simulink model "Project_Model_simulink_version_14_6_2023"  (R2021a)
settings: Solver=FixedStepDiscrete  StartTime=0.0  StopTime=10.0  FixedStep=0.01  RelTol=1e-3
settings Model: Creator=A  LastModifiedBy=A
settings SolverCC: AlgebraicLoopSolver=TrustRegion

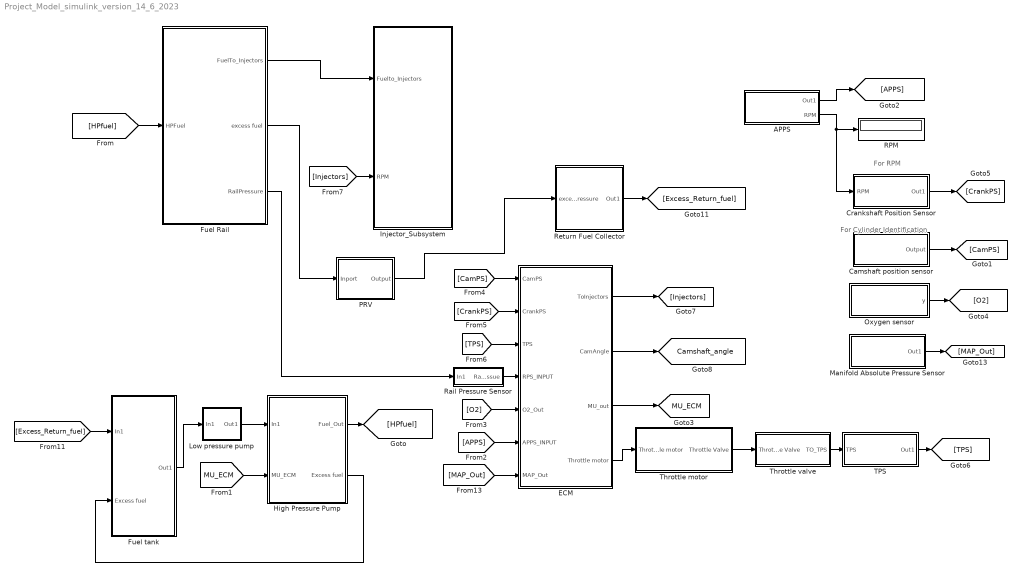
== system Project_Model_simulink_version_14_6_2023 ==
  note: For Cylinder Identification
  note: For RPM
  APPS : Subsystem
  Camshaft position sensor : Subsystem
  Crankshaft Position Sensor : Subsystem
  ECM : Subsystem
  Fuel Rail : Subsystem
  Fuel tank : Subsystem
  High Pressure Pump : Subsystem
  Injector_Subsystem : Subsystem
  Low pressure pump : Subsystem
  Manifold Absolute Pressure Sensor : Subsystem
  Oxygen sensor : Subsystem
  PRV : Subsystem
  RPM : Display
  Rail Pressure Sensor : Subsystem
  Return Fuel Collector : Subsystem
  TPS : Subsystem
  Throttle motor : Subsystem
  Throttle valve : Subsystem
  tag scope: Camshaft_angle=global, MU_ECM=global
  wires:
  Low pressure pump/1(Out1) -> High Pressure Pump/1(In1)
  Fuel tank/1(Out1) -> Low pressure pump/1(In1)
  APPS/1(Out1) -> [APPS]
  [APPS] -> ECM/6(APPS_INPUT)
  ECM/3(MU_out) -> [MU_ECM]
  [O2] -> ECM/5(O2_Out)
  Oxygen sensor/1(y) -> [O2]
  [MU_ECM] -> High Pressure Pump/2(MU_ECM)
  Camshaft position sensor/1(Output) -> [CamPS]
  Fuel Rail/3(RailPressure) -> Rail Pressure Sensor/1(In1)
  Rail Pressure Sensor/1(Rail Pressue) -> ECM/4(RPS_INPUT)
  [CamPS] -> ECM/1(CamPS)
  [CrankPS] -> ECM/2(CrankPS)
  Crankshaft Position Sensor/1(Out1) -> [CrankPS]
  ECM/4(Throttle motor) -> Throttle motor/1(Throttle motor)
  Throttle motor/1(Throttle Valve) -> Throttle valve/1(Throtlle Valve)
  [TPS] -> ECM/3(TPS)
  Fuel Rail/2(excess fuel) -> PRV/1(Inport)
  PRV/1(Output) -> Return Fuel Collector/1(excess rail pressure)
  ECM/1(ToInjectors) -> [Injectors]
  Return Fuel Collector/1(Out1) -> [Excess_Return_fuel]
  [Excess_Return_fuel] -> Fuel tank/1(In1)
  Throttle valve/1(TO_TPS) -> TPS/1(TPS)
  TPS/1(Out1) -> [TPS]
  [MAP_Out] -> ECM/7(MAP_Out)
  Manifold Absolute Pressure Sensor/1(Out1) -> [MAP_Out]
  High Pressure Pump/2(Excess fuel) -> Fuel tank/2(Excess fuel)
  High Pressure Pump/1(Fuel_Out) -> [HPfuel]
  [HPfuel] -> Fuel Rail/1(HPFuel)
  APPS/2(RPM) -> Crankshaft Position Sensor/1(RPM), RPM/1
  Fuel Rail/1(FuelTo_Injectors) -> Injector_Subsystem/1(Fuelto_Injectors)
  [Injectors] -> Injector_Subsystem/2(RPM)
  ECM/2(CamAngle) -> [Camshaft_angle]

== system Project_Model_simulink_version_14_6_2023/APPS ==
  1-D Lookup Table : Lookup_n-D  NumberOfTableDimensions=1  BreakpointsForDimension1=|  BreakpointsForDimension1DataTypeStr=double  Table=|  TableDataTypeStr=double  ExtrapMethod=Clip  InternalRulePriority=Speed  RndMeth=Simplest  InputSameDT=on
      BreakpointsForDimension1=|
      | [8
      | 10
      | 12
      | 14
      | 16
      | 18
      | 20
      | 22
      | 24
      | 26
      | 28
      | 30
      | 32
      | 34
      | 36
      | 38
      | 40
      | 42
      | 44
      | 46
      | 48
      | 50
      | 52
      | 54
      | 56
      | 58
      | 60
      | 62
      | 64
      | 66
      | 68
      | 70
      | 72
      | 74
      | 76
      | 78
      | 80
      | 82
      | 84
      | 86
      | 88
      | 90]
      Table=|
      | [600
      | 730
      | 860
      | 990
      | 1120
      | 1250
      | 1380
      | 1510
      | 1640
      | 1770
      | 1900
      | 2030
      | 2160
      | 2290
      | 2420
      | 2550
      | 2680
      | 2810
      | 2940
      | 3070
      | 3200
      | 3330
      | 3460
      | 3590
      | 3720
      | 3850
      | 3980
      | 4110
      | 4240
      | 4370
      | 4500
      | 4630
      | 4760
      | 4890
      | 5020
      | 5150
      | 5280
      | 5410
      | 5540
      | 5670
      | 5800
      | 6000]
  PedalPositionInDegrees : Constant  Value=11
  Out1 : Outport
  RPM : Outport  Port=2
  tag scope: RPM=global
  wires:
  1-D Lookup Table/1 -> [RPM], RPM/1
  PedalPositionInDegrees/1 -> 1-D Lookup Table/1, Out1/1

== system Project_Model_simulink_version_14_6_2023/Camshaft position sensor ==
  Constant : Constant
  Output : Outport
  wires:
  Constant/1 -> Output/1  "Cam_angle"

== system Project_Model_simulink_version_14_6_2023/Crankshaft Position Sensor ==
  RPM : Inport
  Out1 : Outport
  wires:
  RPM/1 -> Out1/1

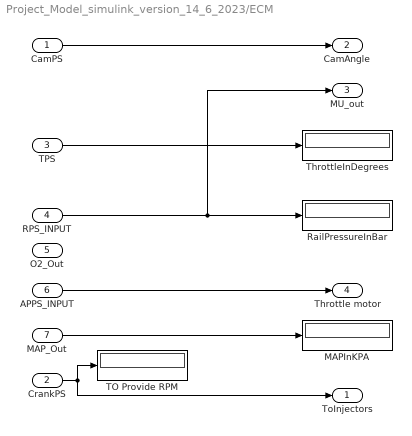
== system Project_Model_simulink_version_14_6_2023/ECM ==
  CamPS : Inport
  CrankPS : Inport  Port=2
  TPS : Inport  Port=3
  RPS_INPUT : Inport  Port=4
  O2_Out : Inport  Port=5
  APPS_INPUT : Inport  Port=6
  MAP_Out : Inport  Port=7
  MAPInKPA : Display
  RailPressureInBar : Display
  TO Provide RPM : Display
  ThrottleInDegrees : Display
  ToInjectors : Outport
  CamAngle : Outport  Port=2
  MU_out : Outport  Port=3
  Throttle motor : Outport  Port=4
  wires:
  CamPS/1 -> CamAngle/1
  APPS_INPUT/1 -> Throttle motor/1
  MAP_Out/1 -> MAPInKPA/1
  TPS/1 -> ThrottleInDegrees/1
  RPS_INPUT/1 -> MU_out/1, RailPressureInBar/1
  CrankPS/1 -> TO Provide RPM/1, ToInjectors/1

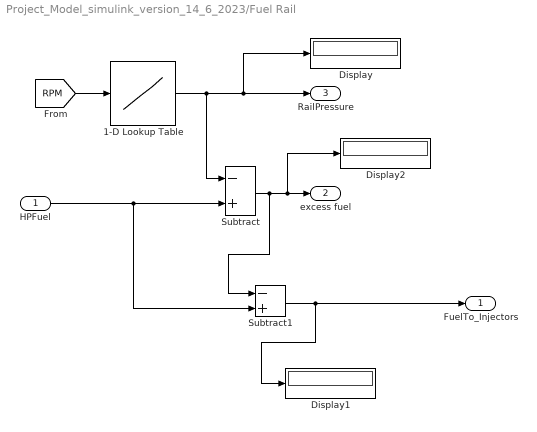
== system Project_Model_simulink_version_14_6_2023/Fuel Rail ==
  HPFuel : Inport
  1-D Lookup Table : Lookup_n-D  NumberOfTableDimensions=1  BreakpointsForDimension1=|  Table=|  InternalRulePriority=Speed  RndMeth=Simplest  InputSameDT=on
      BreakpointsForDimension1=|
      | [600
      | 730
      | 860
      | 990
      | 1120
      | 1250
      | 1380
      | 1510
      | 1640
      | 1770
      | 1900
      | 2030
      | 2160
      | 2290
      | 2420
      | 2550
      | 2680
      | 2810
      | 2940
      | 3070
      | 3200
      | 3330
      | 3460
      | 3590
      | 3720
      | 3850
      | 3980
      | 4110
      | 4240
      | 4370
      | 4500
      | 4630
      | 4760
      | 4890
      | 5020
      | 5150
      | 5280
      | 5410
      | 5540
      | 5670
      | 5800
      | 6000]
      Table=|
      | [300
      | 332
      | 364
      | 396
      | 428
      | 460
      | 492
      | 524
      | 556
      | 588
      | 620
      | 652
      | 684
      | 716
      | 748
      | 780
      | 812
      | 844
      | 876
      | 908
      | 940
      | 972
      | 1004
      | 1036
      | 1068
      | 1100
      | 1132
      | 1164
      | 1196
      | 1228
      | 1260
      | 1292
      | 1324
      | 1356
      | 1388
      | 1420
      | 1452
      | 1484
      | 1516
      | 1548
      | 1580
      | 1600]
  Display : Display
  Display1 : Display
  Display2 : Display
  Subtract : Sum  Inputs=-+
  Subtract1 : Sum  Inputs=-+
  FuelTo_Injectors : Outport
  excess fuel : Outport  Port=2
  RailPressure : Outport  Port=3
  wires:
  1-D Lookup Table/1 -> Subtract/1, Display/1, RailPressure/1
  [RPM] -> 1-D Lookup Table/1
  HPFuel/1 -> Subtract1/2, Subtract/2
  Subtract/1 -> Subtract1/1, Display2/1, excess fuel/1
  Subtract1/1 -> Display1/1, FuelTo_Injectors/1

== system Project_Model_simulink_version_14_6_2023/Fuel tank ==
  In1 : Inport
  Excess fuel : Inport  Port=2
  Constant : Constant
  Out1 : Outport
  wires:
  Constant/1 -> Out1/1

== system Project_Model_simulink_version_14_6_2023/High Pressure Pump ==
  note: rpm=3000
      | rail pressure 902 bar
      | output = 1000 bar
      | difference = 98 bar excess
  In1 : Inport
  MU_ECM : Inport  Port=2
  Display : Display
  Gain : Gain  Gain=160
  Metering Unit : Subsystem
  Fuel_Out : Outport
  Excess fuel : Outport  Port=2
  wires:
  In1/1 -> Gain/1, Display/1
  MU_ECM/1 -> Metering Unit/1(MU_ECM)
  Metering Unit/1(Output) -> Excess fuel/1
  Gain/1 -> Fuel_Out/1

== system Project_Model_simulink_version_14_6_2023/Injector_Subsystem ==
  Fuelto_Injectors : Inport
  RPM : Inport  Port=2
  Injector1 : Subsystem
  Injector2 : Subsystem
  Injector3 : Subsystem
  Injector4 : Subsystem
  wires:
  RPM/1 -> Injector1/1(RPM), Injector2/1(RPM), Injector4/1(RPM), Injector3/1(RPM)
  Fuelto_Injectors/1 -> Injector1/2(HPfuel), Injector2/2(HPfuel), Injector4/2(HPfuel1), Injector3/2(HPfuel)

== system Project_Model_simulink_version_14_6_2023/Low pressure pump ==
  In1 : Inport
  Gain : Gain  Gain=10
  Out1 : Outport
  wires:
  In1/1 -> Gain/1
  Gain/1 -> Out1/1

== system Project_Model_simulink_version_14_6_2023/Manifold Absolute Pressure Sensor ==
  1-D Lookup Table : Lookup_n-D  NumberOfTableDimensions=1  BreakpointsForDimension1=|  Table=|  InternalRulePriority=Speed  RndMeth=Simplest  InputSameDT=on
      BreakpointsForDimension1=|
      | [600
      | 730
      | 860
      | 990
      | 1120
      | 1250
      | 1380
      | 1510
      | 1640
      | 1770
      | 1900
      | 2030
      | 2160
      | 2290
      | 2420
      | 2550
      | 2680
      | 2810
      | 2940
      | 3070
      | 3200
      | 3330
      | 3460
      | 3590
      | 3720
      | 3850
      | 3980
      | 4110
      | 4240
      | 4370
      | 4500
      | 4630
      | 4760
      | 4890
      | 5020
      | 5150
      | 5280
      | 5410
      | 5540
      | 5670
      | 5800
      | 6000]
      Table=|
      | [24
      | 24.2
      | 24.3
      | 24.5
      | 24.6
      | 24.8
      | 24.9
      | 25.1
      | 25.2
      | 25.4
      | 25.5
      | 25.7
      | 25.8
      | 26.0
      | 26.1
      | 26.3
      | 26.4
      | 26.6
      | 26.7
      | 26.9
      | 27.0
      | 27.2
      | 27.3
      | 27.5
      | 27.6
      | 27.8
      | 27.9
      | 28.1
      | 28.2
      | 28.4
      | 28.5
      | 28.7
      | 28.8
      | 29.0
      | 29.1
      | 29.3
      | 29.4
      | 29.5
      | 29.7
      | 29.8
      | 29.9
      | 30]
  Display1 : Display
  Out1 : Outport
  wires:
  1-D Lookup Table/1 -> Out1/1
  [RPM] -> Display1/1, 1-D Lookup Table/1

== system Project_Model_simulink_version_14_6_2023/Oxygen sensor ==
  Constant : Constant
  MATLAB Function : MATLAB Function  TreatAsAtomicUnit=on
  y : Outport
  wires:
  MATLAB Function/1(out) -> y/1
  Constant/1 -> MATLAB Function/1(u)

== system Project_Model_simulink_version_14_6_2023/PRV ==
  Inport : Inport
  Output : Outport
  wires:
  Inport/1 -> Output/1

== system Project_Model_simulink_version_14_6_2023/Rail Pressure Sensor ==
  In1 : Inport
  Rail Pressue : Outport
  wires:
  In1/1 -> Rail Pressue/1

== system Project_Model_simulink_version_14_6_2023/Return Fuel Collector ==
  excess rail pressure : Inport
  Display : Display
  Out1 : Outport
  wires:
  excess rail pressure/1 -> Out1/1, Display/1

== system Project_Model_simulink_version_14_6_2023/TPS ==
  TPS : Inport
  Out1 : Outport
  wires:
  TPS/1 -> Out1/1

== system Project_Model_simulink_version_14_6_2023/Throttle motor ==
  Throttle motor : Inport
  Constant : Constant  Value=pi/3
  Constant1 : Constant
  Integrator : Integrator
  MATLAB Function : MATLAB Function  TreatAsAtomicUnit=on
  Mux : Mux  Inputs=2
  accelerator_pedal : Subsystem
  engine_controll_unit : Subsystem
  feedback_sensor : Subsystem
      settings: PortSchema="{\"entries\":[{\"content\":{\"sides\":[{\"content\":{\"connectorIds\":[\"Out1\"]},\"type\":\"ConnectorPlacement.EquallySpacedRectSide\",\"uuid\":\"fe640009-eb11-44be-8596-49d62a5beec8\"},{\"content\":{\"connectorIds\":[\"In1\"],\"side\":\"RIGHT\"},\"type\":\"ConnectorPlacement.EquallySpacedRectSide\",\"uuid\":\"55096441-78fe-4501-a0f7-12f27b21a046\"},{\"content\":{\"connectorIds\":[],\"side\":\"TOP\"},\"type\":\"ConnectorPlacement.EquallySpacedRectSide\",\"uuid\":\"eb36a32d-1c61-4111-82c5-835a656f9bf6\"}]},\"type\":\"ConnectorPlacement.EquallySpacedConnector\",\"uuid\":\"24611814-9bea-49d8-8ce5-1a9dc2d12b43\"}],\"packageUris\":[\"http://schema.mathworks.com/mf0/Connector/R2020b\"],\"version\":\"1.0\"}"
  throttle_system : Subsystem
  Throttle Valve : Outport
  wires:
  Throttle motor/1 -> Throttle Valve/1
  MATLAB Function/1(y) -> accelerator_pedal/1(angel)
  Mux/1 -> MATLAB Function/1(u)
  engine_controll_unit/1(duty) -> throttle_system/2(duty)
  throttle_system/1(theta) -> feedback_sensor/1(throttle_angle)
  engine_controll_unit/2(direction) -> throttle_system/1(direction)
  Constant1/1 -> Integrator/1
  accelerator_pedal/1(voltage) -> engine_controll_unit/1(pedal_volt)
  feedback_sensor/1(throttle_voltage) -> engine_controll_unit/2(throttle _volt)
  Integrator/1 -> Mux/1
  Constant/1 -> Mux/2

== system Project_Model_simulink_version_14_6_2023/Throttle valve ==
  Throtlle Valve : Inport
  TO_TPS : Outport
  wires:
  Throtlle Valve/1 -> TO_TPS/1

== system Project_Model_simulink_version_14_6_2023/High Pressure Pump/Metering Unit ==
  note: if fuel pressure in rail is as per the required in specific rpm then duty cycle is 15 % if pressure is more duty cylce will increase to 20 % until pressure in rail is as per required
  MU_ECM : Inport
  Output : Outport
  wires:
  MU_ECM/1 -> Output/1

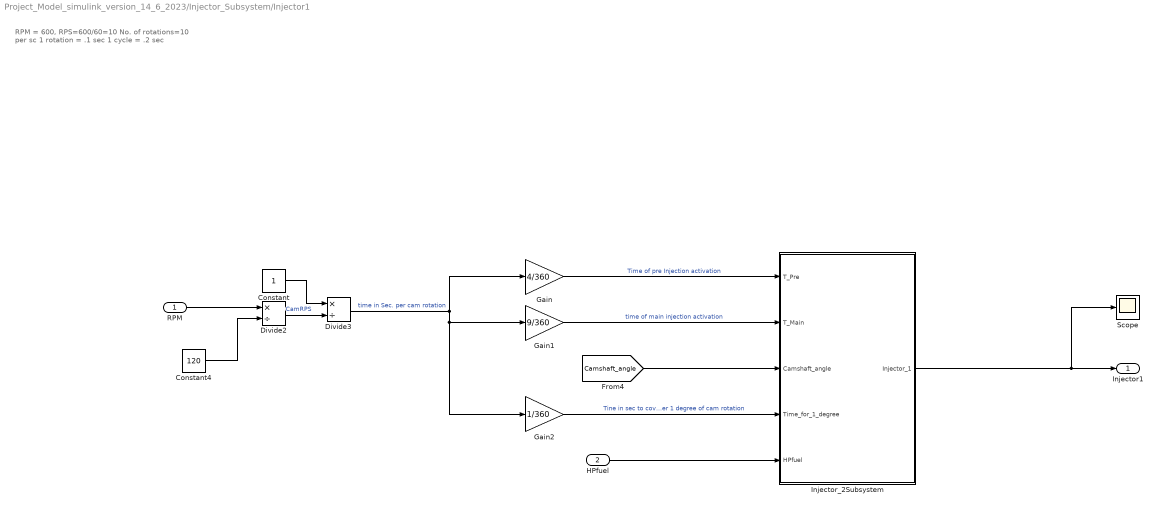
== system Project_Model_simulink_version_14_6_2023/Injector_Subsystem/Injector1 ==
  note: RPM = 600,
      | RPS=600/60=10
      | No. of rotations=10 per sc
      | 1 rotation = .1 sec
      | 1 cycle = .2 sec
  RPM : Inport
  HPfuel : Inport  Port=2
  Constant : Constant
  Constant4 : Constant  Value=120
  Divide2 : Product  Inputs=*/
  Divide3 : Product  Inputs=*/
  Gain : Gain  Gain=4/360
  Gain1 : Gain  Gain=9/360
  Gain2 : Gain  Gain=1/360
  Injector_2Subsystem : Subsystem  TreatAsAtomicUnit=on
  Scope : Scope
  Injector1 : Outport
  wires:
  Gain2/1 -> Injector_2Subsystem/4(Time_for_1_degree)  "Tine in sec to cover 1 degree of cam rotation"
  Gain/1 -> Injector_2Subsystem/1(T_Pre)  "Time of pre Injection activation"
  RPM/1 -> Divide2/1
  Divide3/1 -> Gain/1, Gain2/1, Gain1/1  "time in Sec. per cam rotation"
  Injector_2Subsystem/1(Injector_1) -> Scope/1, Injector1/1
  Divide2/1 -> Divide3/2  "CamRPS"
  [Camshaft_angle] -> Injector_2Subsystem/3(Camshaft_angle)
  HPfuel/1 -> Injector_2Subsystem/5(HPfuel)
  Gain1/1 -> Injector_2Subsystem/2(T_Main)  "time of main injection activation"
  Constant/1 -> Divide3/1
  Constant4/1 -> Divide2/2

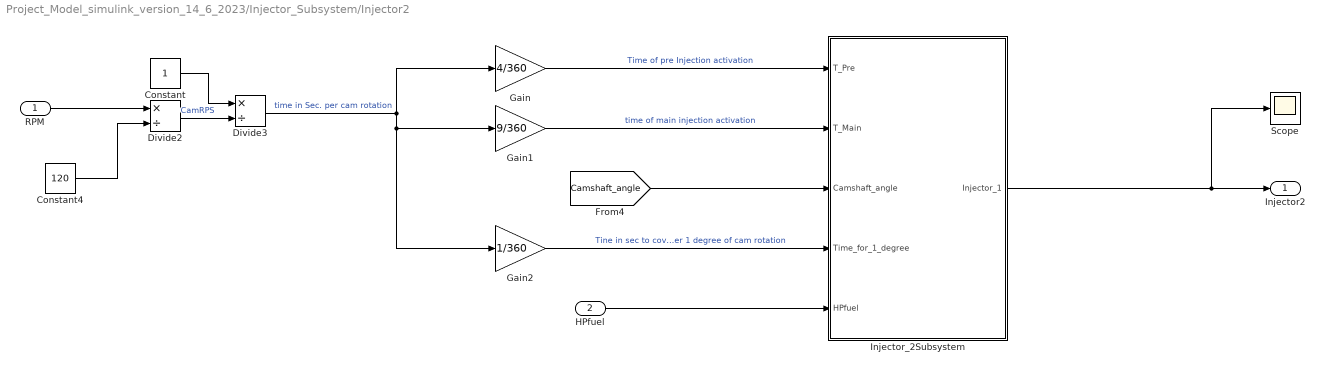
== system Project_Model_simulink_version_14_6_2023/Injector_Subsystem/Injector2 ==
  RPM : Inport
  HPfuel : Inport  Port=2
  Constant : Constant
  Constant4 : Constant  Value=120
  Divide2 : Product  Inputs=*/
  Divide3 : Product  Inputs=*/
  Gain : Gain  Gain=4/360
  Gain1 : Gain  Gain=9/360
  Gain2 : Gain  Gain=1/360
  Injector_2Subsystem : Subsystem  TreatAsAtomicUnit=on
  Scope : Scope
  Injector2 : Outport
  wires:
  Gain2/1 -> Injector_2Subsystem/4(Time_for_1_degree)  "Tine in sec to cover 1 degree of cam rotation"
  Gain/1 -> Injector_2Subsystem/1(T_Pre)  "Time of pre Injection activation"
  RPM/1 -> Divide2/1
  Divide3/1 -> Gain/1, Gain2/1, Gain1/1  "time in Sec. per cam rotation"
  Injector_2Subsystem/1(Injector_1) -> Scope/1, Injector2/1
  Divide2/1 -> Divide3/2  "CamRPS"
  [Camshaft_angle] -> Injector_2Subsystem/3(Camshaft_angle)
  HPfuel/1 -> Injector_2Subsystem/5(HPfuel)
  Gain1/1 -> Injector_2Subsystem/2(T_Main)  "time of main injection activation"
  Constant/1 -> Divide3/1
  Constant4/1 -> Divide2/2

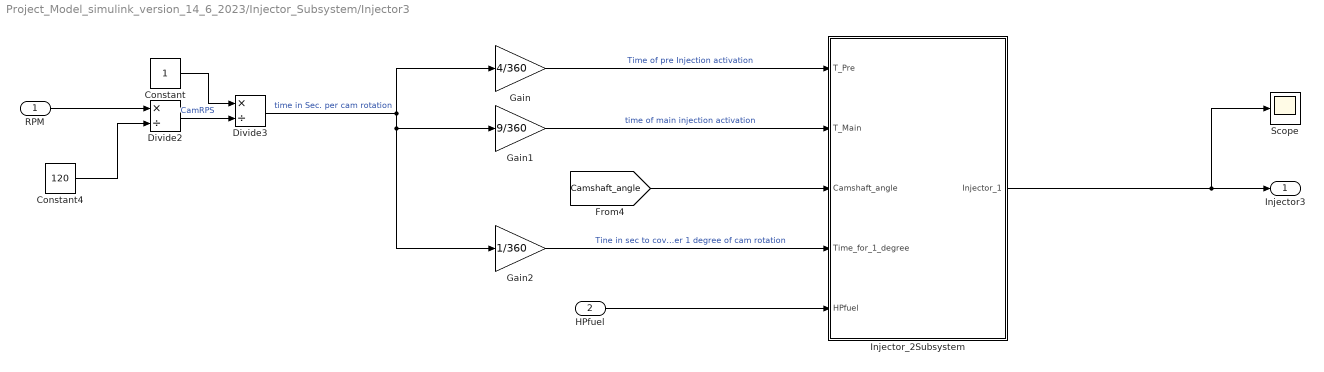
== system Project_Model_simulink_version_14_6_2023/Injector_Subsystem/Injector3 ==
  RPM : Inport
  HPfuel : Inport  Port=2
  Constant : Constant
  Constant4 : Constant  Value=120
  Divide2 : Product  Inputs=*/
  Divide3 : Product  Inputs=*/
  Gain : Gain  Gain=4/360
  Gain1 : Gain  Gain=9/360
  Gain2 : Gain  Gain=1/360
  Injector_2Subsystem : Subsystem  TreatAsAtomicUnit=on
  Scope : Scope
  Injector3 : Outport
  wires:
  Injector_2Subsystem/1(Injector_1) -> Scope/1, Injector3/1
  [Camshaft_angle] -> Injector_2Subsystem/3(Camshaft_angle)
  Gain2/1 -> Injector_2Subsystem/4(Time_for_1_degree)  "Tine in sec to cover 1 degree of cam rotation"
  HPfuel/1 -> Injector_2Subsystem/5(HPfuel)
  Divide3/1 -> Gain/1, Gain2/1, Gain1/1  "time in Sec. per cam rotation"
  Divide2/1 -> Divide3/2  "CamRPS"
  Gain/1 -> Injector_2Subsystem/1(T_Pre)  "Time of pre Injection activation"
  Constant/1 -> Divide3/1
  Constant4/1 -> Divide2/2
  RPM/1 -> Divide2/1
  Gain1/1 -> Injector_2Subsystem/2(T_Main)  "time of main injection activation"

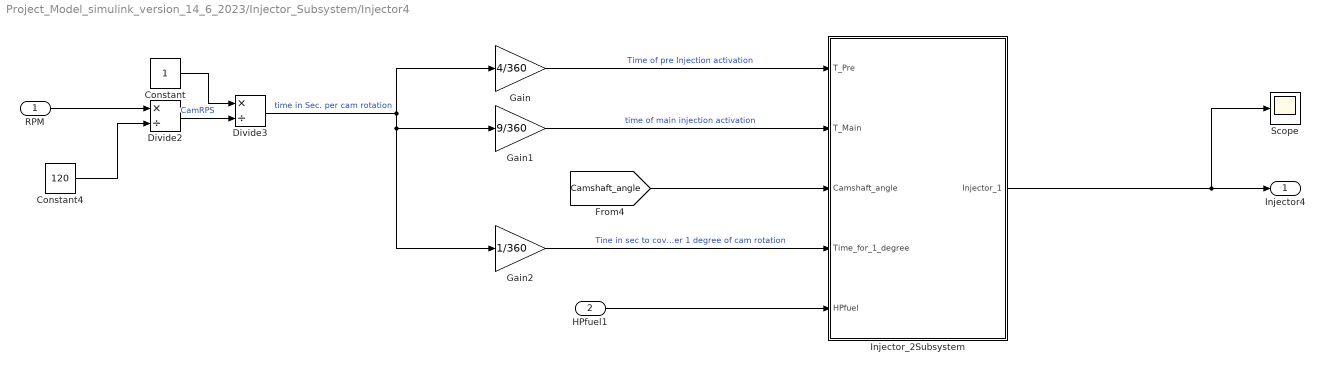
== system Project_Model_simulink_version_14_6_2023/Injector_Subsystem/Injector4 ==
  RPM : Inport
  HPfuel1 : Inport  Port=2
  Constant : Constant
  Constant4 : Constant  Value=120
  Divide2 : Product  Inputs=*/
  Divide3 : Product  Inputs=*/
  Gain : Gain  Gain=4/360
  Gain1 : Gain  Gain=9/360
  Gain2 : Gain  Gain=1/360
  Injector_2Subsystem : Subsystem  TreatAsAtomicUnit=on
  Scope : Scope
  Injector4 : Outport
  wires:
  Gain2/1 -> Injector_2Subsystem/4(Time_for_1_degree)  "Tine in sec to cover 1 degree of cam rotation"
  Gain/1 -> Injector_2Subsystem/1(T_Pre)  "Time of pre Injection activation"
  RPM/1 -> Divide2/1
  Divide3/1 -> Gain/1, Gain2/1, Gain1/1  "time in Sec. per cam rotation"
  Injector_2Subsystem/1(Injector_1) -> Scope/1, Injector4/1
  Divide2/1 -> Divide3/2  "CamRPS"
  [Camshaft_angle] -> Injector_2Subsystem/3(Camshaft_angle)
  HPfuel1/1 -> Injector_2Subsystem/5(HPfuel)
  Gain1/1 -> Injector_2Subsystem/2(T_Main)  "time of main injection activation"
  Constant/1 -> Divide3/1
  Constant4/1 -> Divide2/2

== system Project_Model_simulink_version_14_6_2023/Throttle motor/accelerator_pedal ==
  angel : Inport
  1-D Lookup Table : Lookup_n-D  NumberOfTableDimensions=1  BreakpointsForDimension1=[0 90]  Table=[0.5 4.5]  InternalRulePriority=Speed  RndMeth=Simplest  InputSameDT=on
  Gain : Gain  Gain=180/pi
  voltage : Outport
  wires:
  1-D Lookup Table/1 -> voltage/1
  Gain/1 -> 1-D Lookup Table/1
  angel/1 -> Gain/1

== system Project_Model_simulink_version_14_6_2023/Throttle motor/engine_controll_unit ==
  pedal_volt : Inport
  throttle _volt : Inport  Port=2
  Add : Sum  Inputs=+-
  Subsystem : Subsystem
  duty : Outport
  direction : Outport  Port=2
  wires:
  Add/1 -> Subsystem/1(In1)
  pedal_volt/1 -> Add/1
  throttle _volt/1 -> Add/2
  Subsystem/1(Out1) -> duty/1
  Subsystem/2(Out2) -> direction/1

== system Project_Model_simulink_version_14_6_2023/Throttle motor/feedback_sensor ==
  throttle_angle : Inport
  Subsystem : Subsystem
  throttle_voltage : Outport
  wires:
  throttle_angle/1 -> Subsystem/1(angle)
  Subsystem/1(voltage) -> throttle_voltage/1

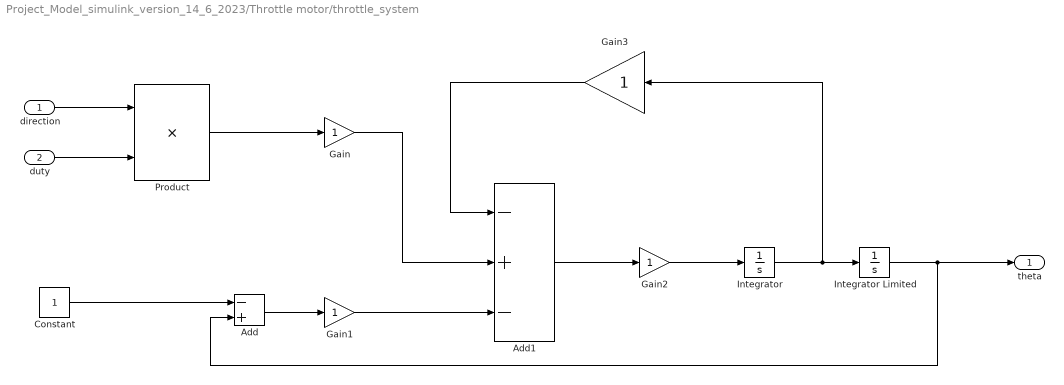
== system Project_Model_simulink_version_14_6_2023/Throttle motor/throttle_system ==
  direction : Inport
  duty : Inport  Port=2
  Add : Sum  Inputs=-+
  Add1 : Sum  Inputs=-+-
  Constant : Constant
  Gain{,1..3} (4 alike) : Gain
  Integrator : Integrator
  Integrator Limited : Integrator  LimitOutput=on  UpperSaturationLimit=pi/2  LowerSaturationLimit=0
  Product : Product
  theta : Outport
  wires:
  direction/1 -> Product/1
  duty/1 -> Product/2
  Product/1 -> Gain/1
  Add/1 -> Gain1/1
  Gain/1 -> Add1/2
  Gain1/1 -> Add1/3
  Constant/1 -> Add/1
  Gain2/1 -> Integrator/1
  Add1/1 -> Gain2/1
  Integrator/1 -> Gain3/1, Integrator Limited/1
  Integrator Limited/1 -> Add/2, theta/1
  Gain3/1 -> Add1/1

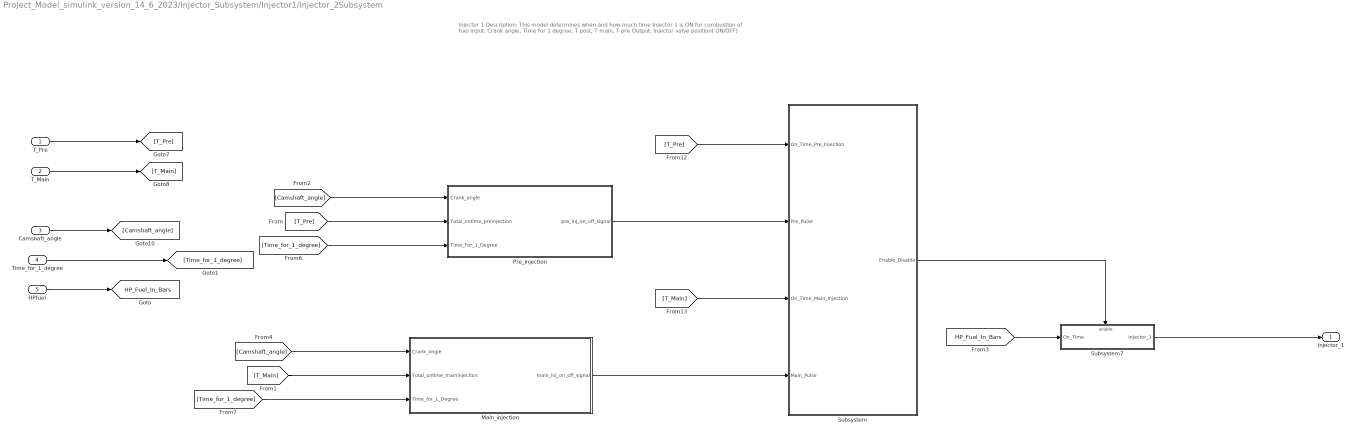
== system Project_Model_simulink_version_14_6_2023/Injector_Subsystem/Injector1/Injector_2Subsystem ==
  note: Injector 1
      | Description: This model determines when and how much time Injector 1 is ON for combustion of fuel
      | Input: Crank angle, TIme for 1 degree, T post, T main, T pre
      | Output: Injector valve position( ON/OFF)
  T_Pre : Inport
  T_Main : Inport  Port=2
  Camshaft_angle : Inport  Port=3
  Time_for_1_degree : Inport  Port=4
  HPfuel : Inport  Port=5
  Main_injection : Subsystem  TreatAsAtomicUnit=on
  Pre_injection : Subsystem  TreatAsAtomicUnit=on
  Subsystem : Subsystem
  Subsystem7 : Subsystem
  Injector_1 : Outport
  tag scope: HP_Fuel_In_Bars=global
  wires:
  T_Pre/1 -> [T_Pre]
  T_Main/1 -> [T_Main]
  Time_for_1_degree/1 -> [Time_for_1_degree]
  [Time_for_1_degree] -> Main_injection/3(Time_for_1_Degree)
  [T_Main] -> Main_injection/2(Total_ontime_maininjection)
  [Camshaft_angle] -> Main_injection/1(Crank_angle)
  [Time_for_1_degree] -> Pre_injection/3(Time_For_1_Degree)
  [Camshaft_angle] -> Pre_injection/1(Crank_angle)
  [T_Pre] -> Pre_injection/2(Total_ontime_preinjection)
  Subsystem/1(Enable_Disable) -> Subsystem7/Enable
  Subsystem7/1(Injector_1) -> Injector_1/1
  [T_Pre] -> Subsystem/1(On_Time_Pre_Injection)
  [T_Main] -> Subsystem/3(On_Time_Main_Injection)
  Main_injection/1(main_inj_on_off_signal) -> Subsystem/4(Main_Pulse)
  Pre_injection/1(pre_inj_on_off_signal) -> Subsystem/2(Pre_Pulse)
  [HP_Fuel_In_Bars] -> Subsystem7/1(On_Time)
  HPfuel/1 -> [HP_Fuel_In_Bars]
  Camshaft_angle/1 -> [Camshaft_angle]

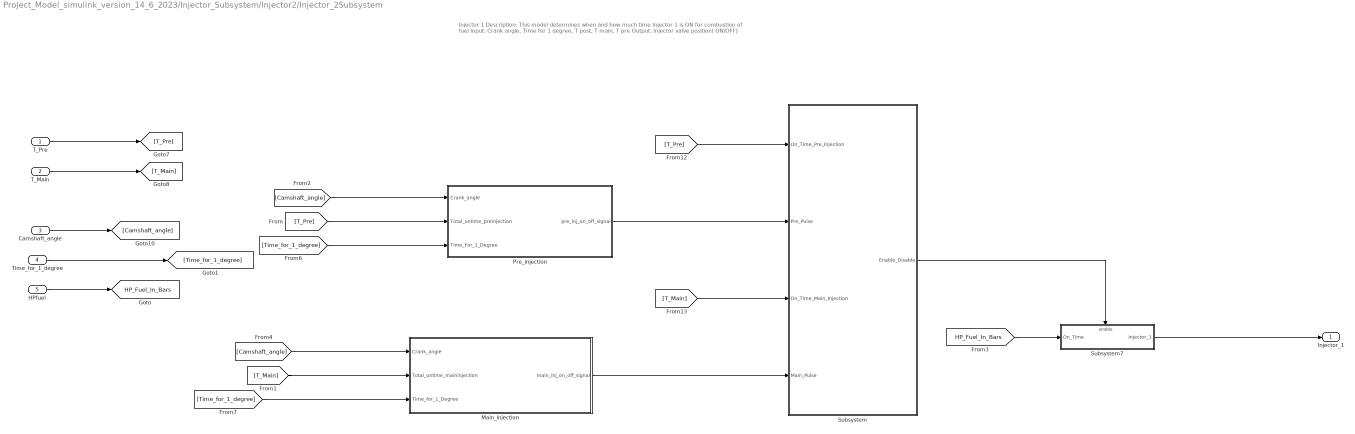
== system Project_Model_simulink_version_14_6_2023/Injector_Subsystem/Injector2/Injector_2Subsystem ==
  note: Injector 1
      | Description: This model determines when and how much time Injector 1 is ON for combustion of fuel
      | Input: Crank angle, TIme for 1 degree, T post, T main, T pre
      | Output: Injector valve position( ON/OFF)
  T_Pre : Inport
  T_Main : Inport  Port=2
  Camshaft_angle : Inport  Port=3
  Time_for_1_degree : Inport  Port=4
  HPfuel : Inport  Port=5
  Main_injection : Subsystem  TreatAsAtomicUnit=on
  Pre_injection : Subsystem  TreatAsAtomicUnit=on
  Subsystem : Subsystem
  Subsystem7 : Subsystem
  Injector_1 : Outport
  tag scope: HP_Fuel_In_Bars=global
  wires:
  T_Pre/1 -> [T_Pre]
  T_Main/1 -> [T_Main]
  Time_for_1_degree/1 -> [Time_for_1_degree]
  [Time_for_1_degree] -> Main_injection/3(Time_for_1_Degree)
  [T_Main] -> Main_injection/2(Total_ontime_maininjection)
  [Camshaft_angle] -> Main_injection/1(Crank_angle)
  [Time_for_1_degree] -> Pre_injection/3(Time_For_1_Degree)
  [Camshaft_angle] -> Pre_injection/1(Crank_angle)
  [T_Pre] -> Pre_injection/2(Total_ontime_preinjection)
  Subsystem/1(Enable_Disable) -> Subsystem7/Enable
  Subsystem7/1(Injector_1) -> Injector_1/1
  [T_Pre] -> Subsystem/1(On_Time_Pre_Injection)
  [T_Main] -> Subsystem/3(On_Time_Main_Injection)
  Main_injection/1(main_inj_on_off_signal) -> Subsystem/4(Main_Pulse)
  Pre_injection/1(pre_inj_on_off_signal) -> Subsystem/2(Pre_Pulse)
  [HP_Fuel_In_Bars] -> Subsystem7/1(On_Time)
  HPfuel/1 -> [HP_Fuel_In_Bars]
  Camshaft_angle/1 -> [Camshaft_angle]

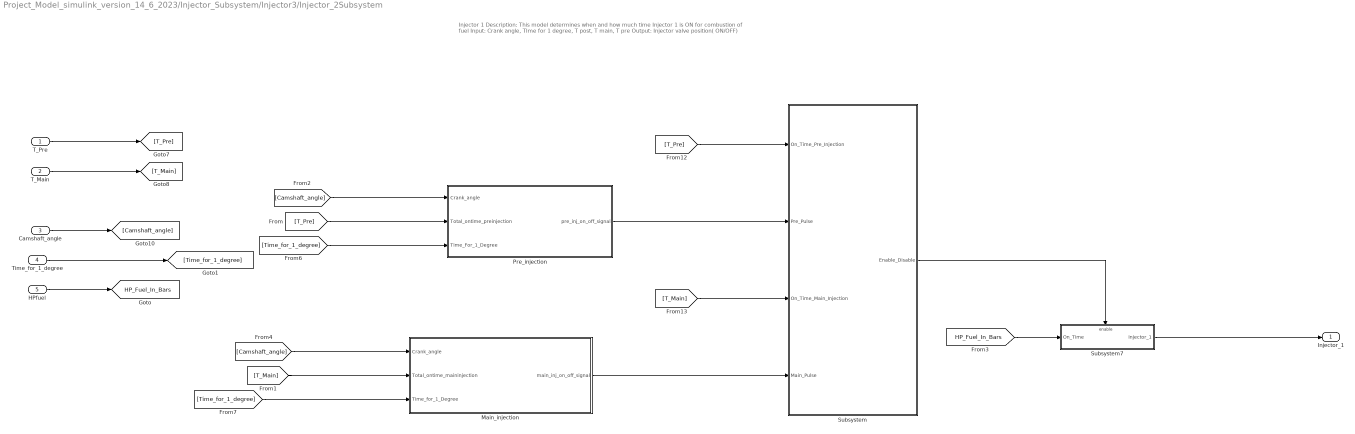
== system Project_Model_simulink_version_14_6_2023/Injector_Subsystem/Injector3/Injector_2Subsystem ==
  note: Injector 1
      | Description: This model determines when and how much time Injector 1 is ON for combustion of fuel
      | Input: Crank angle, TIme for 1 degree, T post, T main, T pre
      | Output: Injector valve position( ON/OFF)
  T_Pre : Inport
  T_Main : Inport  Port=2
  Camshaft_angle : Inport  Port=3
  Time_for_1_degree : Inport  Port=4
  HPfuel : Inport  Port=5
  Main_injection : Subsystem  TreatAsAtomicUnit=on
  Pre_injection : Subsystem  TreatAsAtomicUnit=on
  Subsystem : Subsystem
  Subsystem7 : Subsystem
  Injector_1 : Outport
  tag scope: HP_Fuel_In_Bars=global
  wires:
  T_Pre/1 -> [T_Pre]
  T_Main/1 -> [T_Main]
  Time_for_1_degree/1 -> [Time_for_1_degree]
  [Time_for_1_degree] -> Main_injection/3(Time_for_1_Degree)
  [T_Main] -> Main_injection/2(Total_ontime_maininjection)
  [Camshaft_angle] -> Main_injection/1(Crank_angle)
  [Time_for_1_degree] -> Pre_injection/3(Time_For_1_Degree)
  [Camshaft_angle] -> Pre_injection/1(Crank_angle)
  [T_Pre] -> Pre_injection/2(Total_ontime_preinjection)
  Subsystem/1(Enable_Disable) -> Subsystem7/Enable
  Subsystem7/1(Injector_1) -> Injector_1/1
  [T_Pre] -> Subsystem/1(On_Time_Pre_Injection)
  [T_Main] -> Subsystem/3(On_Time_Main_Injection)
  Main_injection/1(main_inj_on_off_signal) -> Subsystem/4(Main_Pulse)
  Pre_injection/1(pre_inj_on_off_signal) -> Subsystem/2(Pre_Pulse)
  [HP_Fuel_In_Bars] -> Subsystem7/1(On_Time)
  HPfuel/1 -> [HP_Fuel_In_Bars]
  Camshaft_angle/1 -> [Camshaft_angle]

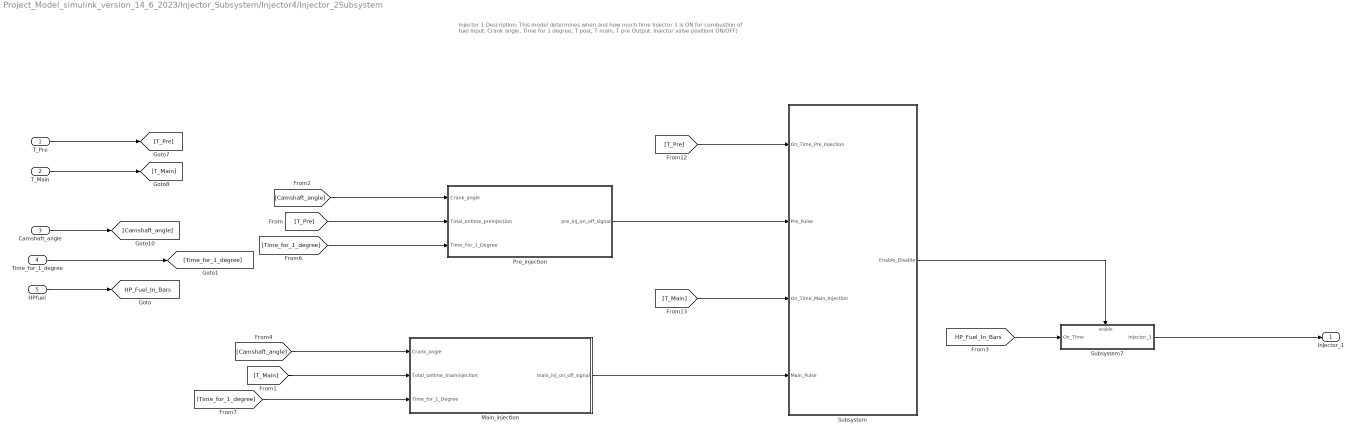
== system Project_Model_simulink_version_14_6_2023/Injector_Subsystem/Injector4/Injector_2Subsystem ==
  note: Injector 1
      | Description: This model determines when and how much time Injector 1 is ON for combustion of fuel
      | Input: Crank angle, TIme for 1 degree, T post, T main, T pre
      | Output: Injector valve position( ON/OFF)
  T_Pre : Inport
  T_Main : Inport  Port=2
  Camshaft_angle : Inport  Port=3
  Time_for_1_degree : Inport  Port=4
  HPfuel : Inport  Port=5
  Main_injection : Subsystem  TreatAsAtomicUnit=on
  Pre_injection : Subsystem  TreatAsAtomicUnit=on
  Subsystem : Subsystem
  Subsystem7 : Subsystem
  Injector_1 : Outport
  tag scope: HP_Fuel_In_Bars=global
  wires:
  T_Pre/1 -> [T_Pre]
  T_Main/1 -> [T_Main]
  Time_for_1_degree/1 -> [Time_for_1_degree]
  [Time_for_1_degree] -> Main_injection/3(Time_for_1_Degree)
  [T_Main] -> Main_injection/2(Total_ontime_maininjection)
  [Camshaft_angle] -> Main_injection/1(Crank_angle)
  [Time_for_1_degree] -> Pre_injection/3(Time_For_1_Degree)
  [Camshaft_angle] -> Pre_injection/1(Crank_angle)
  [T_Pre] -> Pre_injection/2(Total_ontime_preinjection)
  Subsystem/1(Enable_Disable) -> Subsystem7/Enable
  Subsystem7/1(Injector_1) -> Injector_1/1
  [T_Pre] -> Subsystem/1(On_Time_Pre_Injection)
  [T_Main] -> Subsystem/3(On_Time_Main_Injection)
  Main_injection/1(main_inj_on_off_signal) -> Subsystem/4(Main_Pulse)
  Pre_injection/1(pre_inj_on_off_signal) -> Subsystem/2(Pre_Pulse)
  [HP_Fuel_In_Bars] -> Subsystem7/1(On_Time)
  HPfuel/1 -> [HP_Fuel_In_Bars]
  Camshaft_angle/1 -> [Camshaft_angle]

== system Project_Model_simulink_version_14_6_2023/Throttle motor/engine_controll_unit/Subsystem ==
  In1 : Inport
  Abs : Abs
  Constant : Constant
  Constant1 : Constant  Value=-1
  Saturation : Saturate
  Switch : Switch
  Out1 : Outport
  Out2 : Outport  Port=2
  wires:
  Abs/1 -> Saturation/1
  In1/1 -> Switch/2, Abs/1
  Constant/1 -> Switch/1
  Constant1/1 -> Switch/3
  Saturation/1 -> Out1/1
  Switch/1 -> Out2/1

== system Project_Model_simulink_version_14_6_2023/Throttle motor/feedback_sensor/Subsystem ==
  angle : Inport
  1-D Lookup Table : Lookup_n-D  NumberOfTableDimensions=1  BreakpointsForDimension1=[0 90]  Table=[0.5 4.5]  InternalRulePriority=Speed  RndMeth=Simplest  InputSameDT=on
  Gain : Gain  Gain=180/pi
  voltage : Outport
  wires:
  1-D Lookup Table/1 -> voltage/1
  Gain/1 -> 1-D Lookup Table/1
  angle/1 -> Gain/1

== system Project_Model_simulink_version_14_6_2023/Injector_Subsystem/Injector1/Injector_2Subsystem/Main_injection ==
  Crank_angle : Inport  OutDataTypeStr=single
  Total_ontime_maininjection : Inport  Port=2  OutDataTypeStr=single
  Time_for_1_Degree : Inport  Port=3  OutDataTypeStr=single
  Add : Sum  AccumDataTypeStr=single
      settings: AttributesFormatString=AccumDataTypeStr=%<AccumDataTypeStr>
  Divide : Product  Inputs=*/  OutDataTypeStr=single
  Logical Operator : Logic  AllPortsSameDT=off  OutDataTypeStr=boolean
  Main_Inj_trg_angle_inj1 : Constant  Value=180
  Main_Inj_trg_angle_inj2 : Constant  Value=180
  Relational Operator : RelationalOperator  OutDataTypeStr=boolean  RndMeth=Simplest
  Relational Operator1 : RelationalOperator  Operator=<=  OutDataTypeStr=boolean  RndMeth=Simplest
  main_inj_on_off_signal : Outport  VectorParamsAs1DForOutWhenUnconnected=off
  wires:
  Logical Operator/1 -> main_inj_on_off_signal/1  "main_inj_on_off_signal"
  Time_for_1_Degree/1 -> Divide/2
  Relational Operator/1 -> Logical Operator/1
  Main_Inj_trg_angle_inj2/1 -> Add/1
  Add/1 -> Relational Operator1/2  "Total_On_Degree"
  Crank_angle/1 -> Relational Operator1/1, Relational Operator/1
  Main_Inj_trg_angle_inj1/1 -> Relational Operator/2
  Relational Operator1/1 -> Logical Operator/2
  Total_ontime_maininjection/1 -> Divide/1
  Divide/1 -> Add/2

== system Project_Model_simulink_version_14_6_2023/Injector_Subsystem/Injector1/Injector_2Subsystem/Pre_injection ==
  Crank_angle : Inport  OutDataTypeStr=single
  Total_ontime_preinjection : Inport  Port=2  OutDataTypeStr=single
  Time_For_1_Degree : Inport  Port=3  OutDataTypeStr=single
  Add : Sum  AccumDataTypeStr=single
      settings: AttributesFormatString=AccumDataTypeStr=%<AccumDataTypeStr>
  Divide : Product  Inputs=*/  OutDataTypeStr=single
  Logical Operator : Logic  AllPortsSameDT=off  OutDataTypeStr=boolean
  Pre_Inj_trg_angle_inj1 : Constant  Value=175
  Pre_Inj_trg_angle_inj2 : Constant  Value=175
  Relational Operator : RelationalOperator  OutDataTypeStr=boolean  RndMeth=Simplest
  Relational Operator1 : RelationalOperator  Operator=<=  OutDataTypeStr=boolean  RndMeth=Simplest
  pre_inj_on_off_signal : Outport  VectorParamsAs1DForOutWhenUnconnected=off
  wires:
  Divide/1 -> Add/2
  Relational Operator1/1 -> Logical Operator/2
  Pre_Inj_trg_angle_inj1/1 -> Relational Operator/2  "<Trigger_angle>"
  Total_ontime_preinjection/1 -> Divide/1
  Add/1 -> Relational Operator1/2  "Total_On_Degree"
  Pre_Inj_trg_angle_inj2/1 -> Add/1  "<Trigger_angle>"
  Time_For_1_Degree/1 -> Divide/2
  Relational Operator/1 -> Logical Operator/1
  Crank_angle/1 -> Relational Operator1/1, Relational Operator/1
  Logical Operator/1 -> pre_inj_on_off_signal/1  "pre_inj_on_off_signal"

== system Project_Model_simulink_version_14_6_2023/Injector_Subsystem/Injector1/Injector_2Subsystem/Subsystem ==
  note: Subsystem
      | Description: Integrates Pre, Main, Post Injection to single output
      | Input: On time for pre Injection, On time for main Injection, On time for post Injection, Pre Pulse, Main Pulse, Post Pulse
      | Output: On time for Injection
  On_Time_Pre_Injection : Inport
  Pre_Pulse : Inport  Port=2
  On_Time_Main_Injection : Inport  Port=3
  Main_Pulse : Inport  Port=4
  Constant : Constant  Value=0
  Switch1 : Switch  Criteria=u2 ~= 0
  Switch2 : Switch  Criteria=u2 ~= 0
  Enable_Disable : Outport  VectorParamsAs1DForOutWhenUnconnected=off
  wires:
  Main_Pulse/1 -> [main1], Switch2/2
  On_Time_Main_Injection/1 -> Switch2/1
  Pre_Pulse/1 -> Switch1/2, [pre1]
  On_Time_Pre_Injection/1 -> Switch1/1
  Switch1/1 -> Enable_Disable/1  "On_Time_Injection"
  Constant/1 -> Switch2/3  "constant"
  Switch2/1 -> Switch1/3

== system Project_Model_simulink_version_14_6_2023/Injector_Subsystem/Injector1/Injector_2Subsystem/Subsystem7 ==
  note: Pulse for Injector 1
      | Description: Give signal to Injector 1
      | Input: Re rounding constant
      | Output: Pulse to Injector 1
  On_Time : Inport
  Enable : EnablePort  StatesWhenEnabling=reset  PropagateVarSize=During execution
  Injector_1 : Outport  OutDataTypeStr=boolean  VectorParamsAs1DForOutWhenUnconnected=off
  wires:
  On_Time/1 -> Injector_1/1  "HP_fuel_in_Bars"

== system Project_Model_simulink_version_14_6_2023/Injector_Subsystem/Injector2/Injector_2Subsystem/Main_injection ==
  Crank_angle : Inport  OutDataTypeStr=single
  Total_ontime_maininjection : Inport  Port=2  OutDataTypeStr=single
  Time_for_1_Degree : Inport  Port=3  OutDataTypeStr=single
  Add : Sum  AccumDataTypeStr=single
      settings: AttributesFormatString=AccumDataTypeStr=%<AccumDataTypeStr>
  Divide : Product  Inputs=*/  OutDataTypeStr=single
  Logical Operator : Logic  AllPortsSameDT=off  OutDataTypeStr=boolean
  Main_Inj_trg_angle_inj1 : Constant  Value=180
  Main_Inj_trg_angle_inj2 : Constant  Value=180
  Relational Operator : RelationalOperator  OutDataTypeStr=boolean  RndMeth=Simplest
  Relational Operator1 : RelationalOperator  Operator=<=  OutDataTypeStr=boolean  RndMeth=Simplest
  main_inj_on_off_signal : Outport  VectorParamsAs1DForOutWhenUnconnected=off
  wires:
  Logical Operator/1 -> main_inj_on_off_signal/1  "main_inj_on_off_signal"
  Time_for_1_Degree/1 -> Divide/2
  Relational Operator/1 -> Logical Operator/1
  Main_Inj_trg_angle_inj2/1 -> Add/1
  Add/1 -> Relational Operator1/2  "Total_On_Degree"
  Crank_angle/1 -> Relational Operator1/1, Relational Operator/1
  Main_Inj_trg_angle_inj1/1 -> Relational Operator/2
  Relational Operator1/1 -> Logical Operator/2
  Total_ontime_maininjection/1 -> Divide/1
  Divide/1 -> Add/2

== system Project_Model_simulink_version_14_6_2023/Injector_Subsystem/Injector2/Injector_2Subsystem/Pre_injection ==
  Crank_angle : Inport  OutDataTypeStr=single
  Total_ontime_preinjection : Inport  Port=2  OutDataTypeStr=single
  Time_For_1_Degree : Inport  Port=3  OutDataTypeStr=single
  Add : Sum  AccumDataTypeStr=single
      settings: AttributesFormatString=AccumDataTypeStr=%<AccumDataTypeStr>
  Divide : Product  Inputs=*/  OutDataTypeStr=single
  Logical Operator : Logic  AllPortsSameDT=off  OutDataTypeStr=boolean
  Pre_Inj_trg_angle_inj1 : Constant  Value=175
  Pre_Inj_trg_angle_inj2 : Constant  Value=175
  Relational Operator : RelationalOperator  OutDataTypeStr=boolean  RndMeth=Simplest
  Relational Operator1 : RelationalOperator  Operator=<=  OutDataTypeStr=boolean  RndMeth=Simplest
  pre_inj_on_off_signal : Outport  VectorParamsAs1DForOutWhenUnconnected=off
  wires:
  Divide/1 -> Add/2
  Relational Operator1/1 -> Logical Operator/2
  Pre_Inj_trg_angle_inj1/1 -> Relational Operator/2  "<Trigger_angle>"
  Total_ontime_preinjection/1 -> Divide/1
  Add/1 -> Relational Operator1/2  "Total_On_Degree"
  Pre_Inj_trg_angle_inj2/1 -> Add/1  "<Trigger_angle>"
  Time_For_1_Degree/1 -> Divide/2
  Relational Operator/1 -> Logical Operator/1
  Crank_angle/1 -> Relational Operator1/1, Relational Operator/1
  Logical Operator/1 -> pre_inj_on_off_signal/1  "pre_inj_on_off_signal"

== system Project_Model_simulink_version_14_6_2023/Injector_Subsystem/Injector2/Injector_2Subsystem/Subsystem ==
  note: Subsystem
      | Description: Integrates Pre, Main, Post Injection to single output
      | Input: On time for pre Injection, On time for main Injection, On time for post Injection, Pre Pulse, Main Pulse, Post Pulse
      | Output: On time for Injection
  On_Time_Pre_Injection : Inport
  Pre_Pulse : Inport  Port=2
  On_Time_Main_Injection : Inport  Port=3
  Main_Pulse : Inport  Port=4
  Constant : Constant  Value=0
  Switch1 : Switch  Criteria=u2 ~= 0
  Switch2 : Switch  Criteria=u2 ~= 0
  Enable_Disable : Outport  VectorParamsAs1DForOutWhenUnconnected=off
  wires:
  Main_Pulse/1 -> [main1], Switch2/2
  On_Time_Main_Injection/1 -> Switch2/1
  Pre_Pulse/1 -> Switch1/2, [pre1]
  On_Time_Pre_Injection/1 -> Switch1/1
  Switch1/1 -> Enable_Disable/1  "On_Time_Injection"
  Constant/1 -> Switch2/3  "constant"
  Switch2/1 -> Switch1/3

== system Project_Model_simulink_version_14_6_2023/Injector_Subsystem/Injector2/Injector_2Subsystem/Subsystem7 ==
  note: Pulse for Injector 1
      | Description: Give signal to Injector 1
      | Input: Re rounding constant
      | Output: Pulse to Injector 1
  On_Time : Inport
  Enable : EnablePort  StatesWhenEnabling=reset  PropagateVarSize=During execution
  Injector_1 : Outport  OutDataTypeStr=boolean  VectorParamsAs1DForOutWhenUnconnected=off
  wires:
  On_Time/1 -> Injector_1/1  "HP_fuel_in_Bars"

== system Project_Model_simulink_version_14_6_2023/Injector_Subsystem/Injector3/Injector_2Subsystem/Main_injection ==
  Crank_angle : Inport  OutDataTypeStr=single
  Total_ontime_maininjection : Inport  Port=2  OutDataTypeStr=single
  Time_for_1_Degree : Inport  Port=3  OutDataTypeStr=single
  Add : Sum  AccumDataTypeStr=single
      settings: AttributesFormatString=AccumDataTypeStr=%<AccumDataTypeStr>
  Divide : Product  Inputs=*/  OutDataTypeStr=single
  Logical Operator : Logic  AllPortsSameDT=off  OutDataTypeStr=boolean
  Main_Inj_trg_angle_inj1 : Constant  Value=180
  Main_Inj_trg_angle_inj2 : Constant  Value=180
  Relational Operator : RelationalOperator  OutDataTypeStr=boolean  RndMeth=Simplest
  Relational Operator1 : RelationalOperator  Operator=<=  OutDataTypeStr=boolean  RndMeth=Simplest
  main_inj_on_off_signal : Outport  VectorParamsAs1DForOutWhenUnconnected=off
  wires:
  Logical Operator/1 -> main_inj_on_off_signal/1  "main_inj_on_off_signal"
  Time_for_1_Degree/1 -> Divide/2
  Relational Operator/1 -> Logical Operator/1
  Main_Inj_trg_angle_inj2/1 -> Add/1
  Add/1 -> Relational Operator1/2  "Total_On_Degree"
  Crank_angle/1 -> Relational Operator1/1, Relational Operator/1
  Main_Inj_trg_angle_inj1/1 -> Relational Operator/2
  Relational Operator1/1 -> Logical Operator/2
  Total_ontime_maininjection/1 -> Divide/1
  Divide/1 -> Add/2

== system Project_Model_simulink_version_14_6_2023/Injector_Subsystem/Injector3/Injector_2Subsystem/Pre_injection ==
  Crank_angle : Inport  OutDataTypeStr=single
  Total_ontime_preinjection : Inport  Port=2  OutDataTypeStr=single
  Time_For_1_Degree : Inport  Port=3  OutDataTypeStr=single
  Add : Sum  AccumDataTypeStr=single
      settings: AttributesFormatString=AccumDataTypeStr=%<AccumDataTypeStr>
  Divide : Product  Inputs=*/  OutDataTypeStr=single
  Logical Operator : Logic  AllPortsSameDT=off  OutDataTypeStr=boolean
  Pre_Inj_trg_angle_inj1 : Constant  Value=175
  Pre_Inj_trg_angle_inj2 : Constant  Value=175
  Relational Operator : RelationalOperator  OutDataTypeStr=boolean  RndMeth=Simplest
  Relational Operator1 : RelationalOperator  Operator=<=  OutDataTypeStr=boolean  RndMeth=Simplest
  pre_inj_on_off_signal : Outport  VectorParamsAs1DForOutWhenUnconnected=off
  wires:
  Divide/1 -> Add/2
  Relational Operator1/1 -> Logical Operator/2
  Pre_Inj_trg_angle_inj1/1 -> Relational Operator/2  "<Trigger_angle>"
  Total_ontime_preinjection/1 -> Divide/1
  Add/1 -> Relational Operator1/2  "Total_On_Degree"
  Pre_Inj_trg_angle_inj2/1 -> Add/1  "<Trigger_angle>"
  Time_For_1_Degree/1 -> Divide/2
  Relational Operator/1 -> Logical Operator/1
  Crank_angle/1 -> Relational Operator1/1, Relational Operator/1
  Logical Operator/1 -> pre_inj_on_off_signal/1  "pre_inj_on_off_signal"

== system Project_Model_simulink_version_14_6_2023/Injector_Subsystem/Injector3/Injector_2Subsystem/Subsystem ==
  note: Subsystem
      | Description: Integrates Pre, Main, Post Injection to single output
      | Input: On time for pre Injection, On time for main Injection, On time for post Injection, Pre Pulse, Main Pulse, Post Pulse
      | Output: On time for Injection
  On_Time_Pre_Injection : Inport
  Pre_Pulse : Inport  Port=2
  On_Time_Main_Injection : Inport  Port=3
  Main_Pulse : Inport  Port=4
  Constant : Constant  Value=0
  Switch1 : Switch  Criteria=u2 ~= 0
  Switch2 : Switch  Criteria=u2 ~= 0
  Enable_Disable : Outport  VectorParamsAs1DForOutWhenUnconnected=off
  wires:
  Main_Pulse/1 -> [main1], Switch2/2
  On_Time_Main_Injection/1 -> Switch2/1
  Pre_Pulse/1 -> Switch1/2, [pre1]
  On_Time_Pre_Injection/1 -> Switch1/1
  Switch1/1 -> Enable_Disable/1  "On_Time_Injection"
  Constant/1 -> Switch2/3  "constant"
  Switch2/1 -> Switch1/3

== system Project_Model_simulink_version_14_6_2023/Injector_Subsystem/Injector3/Injector_2Subsystem/Subsystem7 ==
  note: Pulse for Injector 1
      | Description: Give signal to Injector 1
      | Input: Re rounding constant
      | Output: Pulse to Injector 1
  On_Time : Inport
  Enable : EnablePort  StatesWhenEnabling=reset  PropagateVarSize=During execution
  Injector_1 : Outport  OutDataTypeStr=boolean  VectorParamsAs1DForOutWhenUnconnected=off
  wires:
  On_Time/1 -> Injector_1/1  "HP_fuel_in_Bars"

== system Project_Model_simulink_version_14_6_2023/Injector_Subsystem/Injector4/Injector_2Subsystem/Main_injection ==
  Crank_angle : Inport  OutDataTypeStr=single
  Total_ontime_maininjection : Inport  Port=2  OutDataTypeStr=single
  Time_for_1_Degree : Inport  Port=3  OutDataTypeStr=single
  Add : Sum  AccumDataTypeStr=single
      settings: AttributesFormatString=AccumDataTypeStr=%<AccumDataTypeStr>
  Divide : Product  Inputs=*/  OutDataTypeStr=single
  Logical Operator : Logic  AllPortsSameDT=off  OutDataTypeStr=boolean
  Main_Inj_trg_angle_inj1 : Constant  Value=180
  Main_Inj_trg_angle_inj2 : Constant  Value=180
  Relational Operator : RelationalOperator  OutDataTypeStr=boolean  RndMeth=Simplest
  Relational Operator1 : RelationalOperator  Operator=<=  OutDataTypeStr=boolean  RndMeth=Simplest
  main_inj_on_off_signal : Outport  VectorParamsAs1DForOutWhenUnconnected=off
  wires:
  Logical Operator/1 -> main_inj_on_off_signal/1  "main_inj_on_off_signal"
  Time_for_1_Degree/1 -> Divide/2
  Relational Operator/1 -> Logical Operator/1
  Main_Inj_trg_angle_inj2/1 -> Add/1
  Add/1 -> Relational Operator1/2  "Total_On_Degree"
  Crank_angle/1 -> Relational Operator1/1, Relational Operator/1
  Main_Inj_trg_angle_inj1/1 -> Relational Operator/2
  Relational Operator1/1 -> Logical Operator/2
  Total_ontime_maininjection/1 -> Divide/1
  Divide/1 -> Add/2

== system Project_Model_simulink_version_14_6_2023/Injector_Subsystem/Injector4/Injector_2Subsystem/Pre_injection ==
  Crank_angle : Inport  OutDataTypeStr=single
  Total_ontime_preinjection : Inport  Port=2  OutDataTypeStr=single
  Time_For_1_Degree : Inport  Port=3  OutDataTypeStr=single
  Add : Sum  AccumDataTypeStr=single
      settings: AttributesFormatString=AccumDataTypeStr=%<AccumDataTypeStr>
  Divide : Product  Inputs=*/  OutDataTypeStr=single
  Logical Operator : Logic  AllPortsSameDT=off  OutDataTypeStr=boolean
  Pre_Inj_trg_angle_inj1 : Constant  Value=175
  Pre_Inj_trg_angle_inj2 : Constant  Value=175
  Relational Operator : RelationalOperator  OutDataTypeStr=boolean  RndMeth=Simplest
  Relational Operator1 : RelationalOperator  Operator=<=  OutDataTypeStr=boolean  RndMeth=Simplest
  pre_inj_on_off_signal : Outport  VectorParamsAs1DForOutWhenUnconnected=off
  wires:
  Divide/1 -> Add/2
  Relational Operator1/1 -> Logical Operator/2
  Pre_Inj_trg_angle_inj1/1 -> Relational Operator/2  "<Trigger_angle>"
  Total_ontime_preinjection/1 -> Divide/1
  Add/1 -> Relational Operator1/2  "Total_On_Degree"
  Pre_Inj_trg_angle_inj2/1 -> Add/1  "<Trigger_angle>"
  Time_For_1_Degree/1 -> Divide/2
  Relational Operator/1 -> Logical Operator/1
  Crank_angle/1 -> Relational Operator1/1, Relational Operator/1
  Logical Operator/1 -> pre_inj_on_off_signal/1  "pre_inj_on_off_signal"

== system Project_Model_simulink_version_14_6_2023/Injector_Subsystem/Injector4/Injector_2Subsystem/Subsystem ==
  note: Subsystem
      | Description: Integrates Pre, Main, Post Injection to single output
      | Input: On time for pre Injection, On time for main Injection, On time for post Injection, Pre Pulse, Main Pulse, Post Pulse
      | Output: On time for Injection
  On_Time_Pre_Injection : Inport
  Pre_Pulse : Inport  Port=2
  On_Time_Main_Injection : Inport  Port=3
  Main_Pulse : Inport  Port=4
  Constant : Constant  Value=0
  Switch1 : Switch  Criteria=u2 ~= 0
  Switch2 : Switch  Criteria=u2 ~= 0
  Enable_Disable : Outport  VectorParamsAs1DForOutWhenUnconnected=off
  wires:
  Main_Pulse/1 -> [main1], Switch2/2
  On_Time_Main_Injection/1 -> Switch2/1
  Pre_Pulse/1 -> Switch1/2, [pre1]
  On_Time_Pre_Injection/1 -> Switch1/1
  Switch1/1 -> Enable_Disable/1  "On_Time_Injection"
  Constant/1 -> Switch2/3  "constant"
  Switch2/1 -> Switch1/3

== system Project_Model_simulink_version_14_6_2023/Injector_Subsystem/Injector4/Injector_2Subsystem/Subsystem7 ==
  note: Pulse for Injector 1
      | Description: Give signal to Injector 1
      | Input: Re rounding constant
      | Output: Pulse to Injector 1
  On_Time : Inport
  Enable : EnablePort  StatesWhenEnabling=reset  PropagateVarSize=During execution
  Injector_1 : Outport  OutDataTypeStr=boolean  VectorParamsAs1DForOutWhenUnconnected=off
  wires:
  On_Time/1 -> Injector_1/1  "HP_fuel_in_Bars"

== matlab function Project_Model_simulink_version_14_6_2023/Oxygen sensor/MATLAB Function ==
  data: u input; out output
function out = fcn(u)
%#codegen

if (u>0.65)
y = 0.95;
elseif (u<=0.65 && u>=0.25)
    y = 1;
else
    y=1.05;
end

out=y;

== matlab function Project_Model_simulink_version_14_6_2023/Throttle motor/MATLAB Function ==
  data: u input; y output
function y = fcn(u)

y = u;
